simulink model "s4dot2_14subsystem"  (R2023b)
settings: Solver=FixedStepAuto  StartTime=0.0  StopTime=10.0  FixedStep=0.25  RelTol=1e-3
settings Model: Creator=lxj  LastModifiedBy=lxj

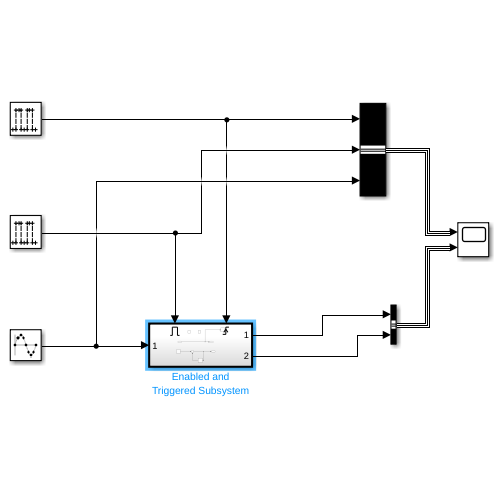
[thumbnail: Simulink's stored preview of the top-level diagram]
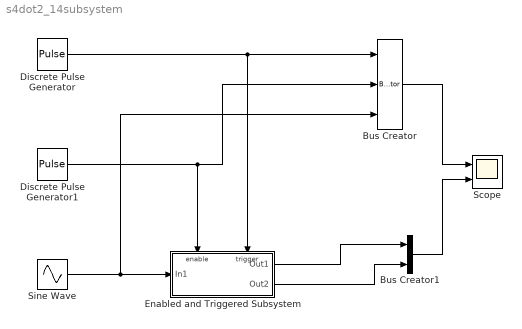
== system s4dot2_14subsystem ==
  Bus Creator : BusCreator  Inputs=3
  Bus Creator1 : BusCreator  Inputs=2
  Discrete Pulse Generator : DiscretePulseGenerator  SampleTime=0.25
  Discrete Pulse Generator1 : DiscretePulseGenerator  Period=20  PulseWidth=10  SampleTime=0.25
  Enabled and Triggered Subsystem : Subsystem  TreatAsAtomicUnit=on
  Scope : Scope  NumInputPorts=2
  Sine Wave : Sin  SineType=Sample based  Samples=20  SampleTime=0.25
  wires:
  Bus Creator/1 -> Scope/1
  Bus Creator1/1 -> Scope/2
  Discrete Pulse Generator/1 -> Enabled and Triggered Subsystem/Trigger, Bus Creator/1
  Discrete Pulse Generator1/1 -> Enabled and Triggered Subsystem/Enable, Bus Creator/2
  Sine Wave/1 -> Enabled and Triggered Subsystem/1(In1), Bus Creator/3
  Enabled and Triggered Subsystem/1(Out1) -> Bus Creator1/1
  Enabled and Triggered Subsystem/2(Out2) -> Bus Creator1/2

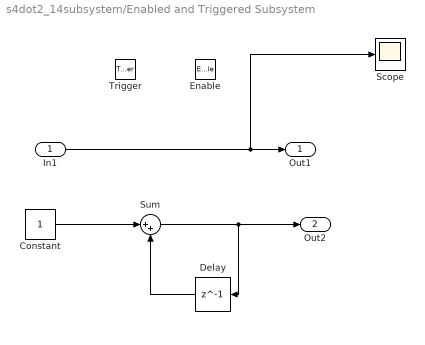
== system s4dot2_14subsystem/Enabled and Triggered Subsystem ==
  In1 : Inport
  Enable : EnablePort
  Trigger : TriggerPort  VariantControl=(inherit)
  Constant : Constant
  Delay : Delay  DelayLength=1  InitialCondition=0
  Scope : Scope
  Sum : Sum  Inputs=|++
  Out1 : Outport  InitialOutput=1
  Out2 : Outport  Port=2  OutputWhenDisabled=reset  InitialOutput=0
  wires:
  In1/1 -> Scope/1, Out1/1
  Constant/1 -> Sum/1
  Sum/1 -> Delay/1, Out2/1
  Delay/1 -> Sum/2
